simulink model "Li_ion_BatteryPack_Model"  (R2022a)
settings: Solver=VariableStepAuto  StartTime=0.0  StopTime=350  RelTol=1e-3
values from neighbouring files (symbols this model uses):
  A = [0 0 0 ... (first row only)    [Lithium_ion_oneCell_Modeling_continuous_Linear.m]    (also in Lithium_ion_oneCell_Modeling_continuous_new.m)
  A_pack = [A1 zeros(3,9);zeros(3,3) A2 zeros(3,6);zeros(3,6) A3 zeros(3,3);zeros(3,9) A4]    [Lithium_ion_oneCell_Modeling_continuous_new.m]
  A_pack_d = sys_d_pack.A    [Lithium_ion_oneCell_Modeling_continuous_new.m]
  B = [-eta/C_max ... (first row only)    [Lithium_ion_oneCell_Modeling_continuous_Linear.m]    (also in Lithium_ion_oneCell_Modeling_continuous_new.m)
  B_pack = [B1;B2;B3;B4]    [Lithium_ion_oneCell_Modeling_continuous_new.m]
  B_pack_d = sys_d_pack.B    [Lithium_ion_oneCell_Modeling_continuous_new.m]
  R0 = 43e-3    (= 0.043)    [Lithium_ion_oneCell_Modeling_continuous_Linear.m]    (also in Lithium_ion_oneCell_Modeling_continuous_new.m)
  R0_pack = [R0;R0;R0;R0]    [Lithium_ion_oneCell_Modeling_continuous_new.m]
  X10 = [0.6;0;0]    [Lithium_ion_oneCell_Modeling_continuous_new.m]
  Zeta0 = [X10;X20;X30;X40]    [Lithium_ion_oneCell_Modeling_continuous_new.m]
undefined symbols (not defined in the file or in its folder): sigbuilder_block
settings Model: Creator=Asus  LastModifiedBy=Asus

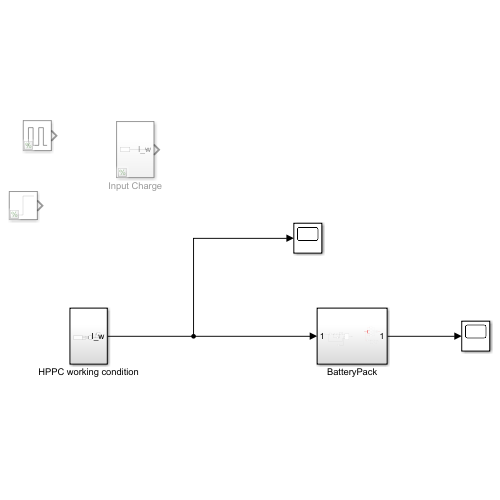
[thumbnail: Simulink's stored preview of the top-level diagram]
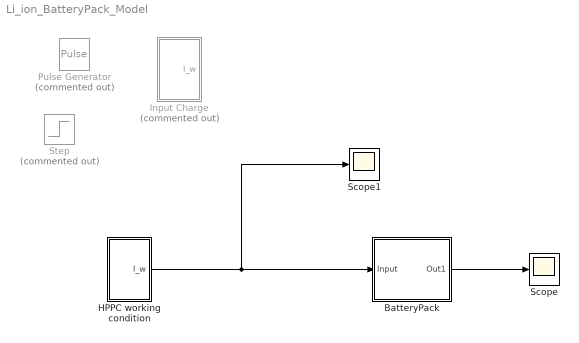
== system Li_ion_BatteryPack_Model ==
  BatteryPack : Subsystem
  HPPC working condition : Subsystem
  Input Charge : Subsystem  Commented=on
  Pulse Generator : DiscretePulseGenerator  Commented=on  PulseType=Time based  Amplitude=-2.4  Period=0.05  PulseWidth=99
  Scope : Scope
  Scope1 : Scope
  Step : Step  Commented=on  Time=10000  Before=-1.2  After=-1.2  SampleTime=0
  wires:
  HPPC working condition/1(I_w) -> Scope1/1, BatteryPack/1(Input)
  BatteryPack/1(Out1) -> Scope/1

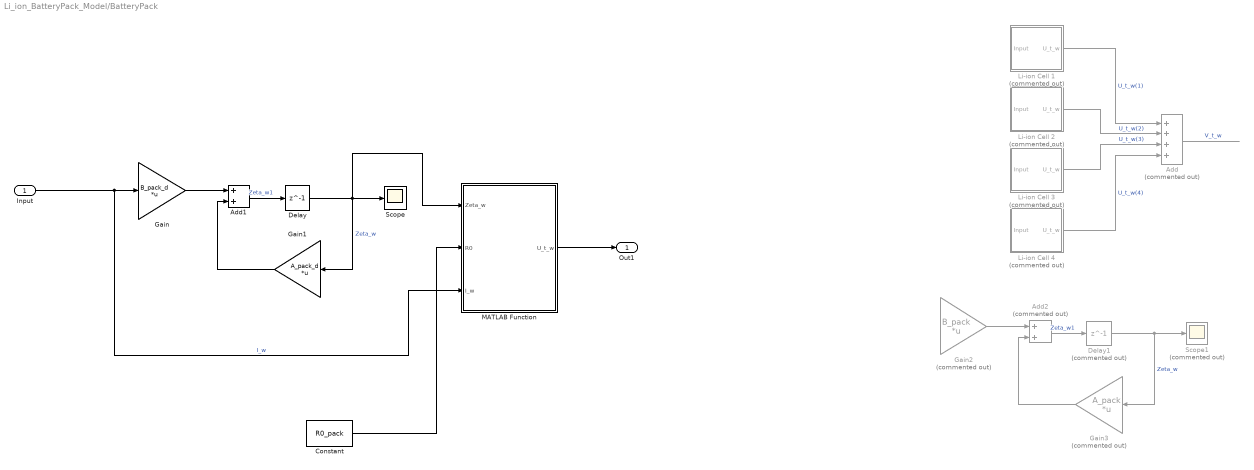
== system Li_ion_BatteryPack_Model/BatteryPack ==
  Input : Inport
  Add : Sum  Commented=on  Inputs=++++
  Add1 : Sum
  Add2 : Sum  Commented=on
  Constant : Constant  Value=R0_pack
  Delay : Delay  DelayLength=1  InitialCondition=Zeta0
  Delay1 : Delay  Commented=on  DelayLength=1  InitialCondition=Zeta0
  Gain : Gain  Gain=B_pack_d  Multiplication=Matrix(K*u)
  Gain1 : Gain  Gain=A_pack_d  Multiplication=Matrix(K*u)
  Gain2 : Gain  Commented=on  Gain=B_pack  Multiplication=Matrix(K*u)
  Gain3 : Gain  Commented=on  Gain=A_pack  Multiplication=Matrix(K*u)
  Li-ion Cell 1 : Subsystem  Commented=on
  Li-ion Cell 2 : Subsystem  Commented=on
  Li-ion Cell 3 : Subsystem  Commented=on
  Li-ion Cell 4 : Subsystem  Commented=on
  MATLAB Function : MATLAB Function  TreatAsAtomicUnit=on
  Scope : Scope
  Scope1 : Scope  Commented=on
  Out1 : Outport
  wires:
  Input/1 -> MATLAB Function/3(I_w), Gain/1  "I_w"
  Gain/1 -> Add1/1
  Add1/1 -> Delay/1  "Zeta_w1"
  Gain1/1 -> Add1/2
  Delay/1 -> Gain1/1, MATLAB Function/1(Zeta_w), Scope/1  "Zeta_w"
  Constant/1 -> MATLAB Function/2(R0)
  MATLAB Function/1(U_t_w) -> Out1/1
  Gain2/1 -> Add2/1
  Delay1/1 -> Scope1/1, Gain3/1  "Zeta_w"
  Li-ion Cell 4/1(U_t_w) -> Add/4  "U_t_w(4)"
  Li-ion Cell 3/1(U_t_w) -> Add/3  "U_t_w(3)"
  Gain3/1 -> Add2/2
  Li-ion Cell 1/1(U_t_w) -> Add/1  "U_t_w(1)"
  ? -> Gain2/1, Li-ion Cell 2/1(Input), Li-ion Cell 1/1(Input), Li-ion Cell 4/1(Input), Li-ion Cell 3/1(Input)  "I_w"
  Li-ion Cell 2/1(U_t_w) -> Add/2  "U_t_w(2)"
  Add/1 -> ?  "V_t_w"
  Add2/1 -> Delay1/1  "Zeta_w1"

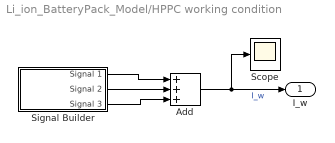
== system Li_ion_BatteryPack_Model/HPPC working condition ==
  Add : Sum  Inputs=+++
  Scope : Scope
  Signal Builder : Subsystem  Tag=STV Subsys  LoadFcn=sigbuilder_block('load');  StartFcn=sigbuilder_block('start');  StopFcn=sigbuilder_block('stop');  ClipboardFcn=sigbuilder_block('clipboard');  mask(Sigbuilder block){tuvar=[0:10]}
      mask help: Simulink:masks:SigbuilderBlock_MD
      mask init:
      | if ~strcmp(get_param(bdroot(gcbh),'SimulationStatus'),'stopped') tuvar = sigbuilder_block('maskInit'); end
      settings: CopyFcn=sigbuilder_block('copy');  DeleteFcn=sigbuilder_block('delete');  ModelCloseFcn=sigbuilder_block('modelClose');  PreSaveFcn=sigbuilder_block('preSave');  PauseFcn=sigbuilder_block('pause');  ContinueFcn=sigbuilder_block('continue');  NameChangeFcn=sigbuilder_block('namechange');  OpenFcn=sigbuilder_block('open',[5.4 36 1141.2 516.6 ]);  CloseFcn=sigbuilder_block('close');
      mask Display: plot(0, 0, 100, 100,[2, 2, 32, 32, 2], [68, 8, 8, 68, 68],[32, 2], [38, 38], [32, 19, 2],[53, 60, 44], [32, 17, 17, 2],[16, 16, 31, 31]);txt = getActiveGroup(gcbh);text(2, 100, txt,'verticalAlignment', 'top');
  I_w : Outport
  wires:
  Add/1 -> Scope/1, I_w/1  "I_w"
  Signal Builder/2(Signal 2) -> Add/2
  Signal Builder/1(Signal 1) -> Add/1
  Signal Builder/3(Signal 3) -> Add/3

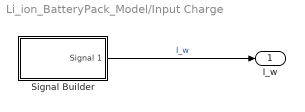
== system Li_ion_BatteryPack_Model/Input Charge ==
  Signal Builder : Subsystem  Tag=STV Subsys  LoadFcn=sigbuilder_block('load');  StartFcn=sigbuilder_block('start');  StopFcn=sigbuilder_block('stop');  ClipboardFcn=sigbuilder_block('clipboard');  mask(Sigbuilder block){tuvar=[0:10]}
      mask help: Simulink:masks:SigbuilderBlock_MD
      mask init:
      | if ~strcmp(get_param(bdroot(gcbh),'SimulationStatus'),'stopped') tuvar = sigbuilder_block('maskInit'); end
      settings: CopyFcn=sigbuilder_block('copy');  DeleteFcn=sigbuilder_block('delete');  ModelCloseFcn=sigbuilder_block('modelClose');  PreSaveFcn=sigbuilder_block('preSave');  PauseFcn=sigbuilder_block('pause');  ContinueFcn=sigbuilder_block('continue');  NameChangeFcn=sigbuilder_block('namechange');  OpenFcn=sigbuilder_block('open',[5.4 36 1141.2 516.6 ]);  CloseFcn=sigbuilder_block('close');
      mask Display: plot(0, 0, 100, 100,[2, 2, 32, 32, 2], [68, 8, 8, 68, 68],[32, 2], [38, 38], [32, 19, 2],[53, 60, 44], [32, 17, 17, 2],[16, 16, 31, 31]);txt = getActiveGroup(gcbh);text(2, 100, txt,'verticalAlignment', 'top');
  I_w : Outport
  wires:
  Signal Builder/1(Signal 1) -> I_w/1  "I_w"

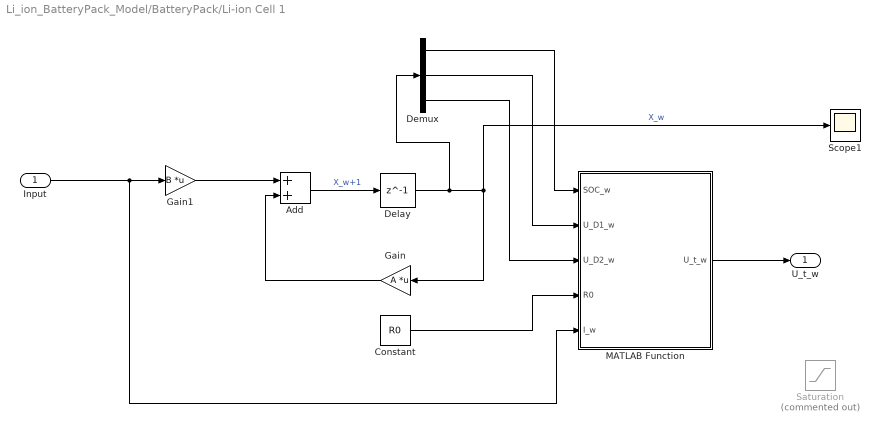
== system Li_ion_BatteryPack_Model/BatteryPack/Li-ion Cell 1 ==
  Input : Inport
  Add : Sum
  Constant : Constant  Value=R0
  Delay : Delay  DelayLength=1  InitialCondition=X10
  Demux : Demux  Outputs=3
  Gain : Gain  Gain=A  Multiplication=Matrix(K*u)
  Gain1 : Gain  Gain=B  Multiplication=Matrix(K*u)
  MATLAB Function : MATLAB Function  TreatAsAtomicUnit=on
  Saturation : Saturate  Commented=on  UpperLimit=4.2  LowerLimit=3
  Scope1 : Scope
  U_t_w : Outport
  wires:
  Input/1 -> MATLAB Function/5(I_w), Gain1/1
  Add/1 -> Delay/1  "X_w+1"
  Demux/1 -> MATLAB Function/1(SOC_w)
  Delay/1 -> Demux/1, Gain/1, Scope1/1  "X_w"
  Gain1/1 -> Add/1
  Demux/3 -> MATLAB Function/3(U_D2_w)
  Gain/1 -> Add/2
  Demux/2 -> MATLAB Function/2(U_D1_w)
  Constant/1 -> MATLAB Function/4(R0)
  MATLAB Function/1(U_t_w) -> U_t_w/1

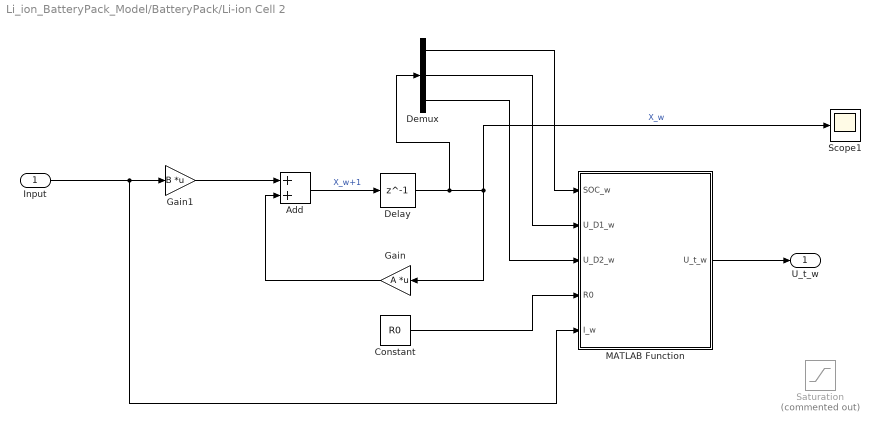
== system Li_ion_BatteryPack_Model/BatteryPack/Li-ion Cell 2 ==
  Input : Inport
  Add : Sum
  Constant : Constant  Value=R0
  Delay : Delay  DelayLength=1  InitialCondition=X10
  Demux : Demux  Outputs=3
  Gain : Gain  Gain=A  Multiplication=Matrix(K*u)
  Gain1 : Gain  Gain=B  Multiplication=Matrix(K*u)
  MATLAB Function : MATLAB Function  TreatAsAtomicUnit=on
  Saturation : Saturate  Commented=on  UpperLimit=4.2  LowerLimit=3
  Scope1 : Scope
  U_t_w : Outport
  wires:
  Input/1 -> MATLAB Function/5(I_w), Gain1/1
  Add/1 -> Delay/1  "X_w+1"
  Demux/1 -> MATLAB Function/1(SOC_w)
  Delay/1 -> Demux/1, Gain/1, Scope1/1  "X_w"
  Gain1/1 -> Add/1
  Demux/3 -> MATLAB Function/3(U_D2_w)
  Gain/1 -> Add/2
  Demux/2 -> MATLAB Function/2(U_D1_w)
  Constant/1 -> MATLAB Function/4(R0)
  MATLAB Function/1(U_t_w) -> U_t_w/1

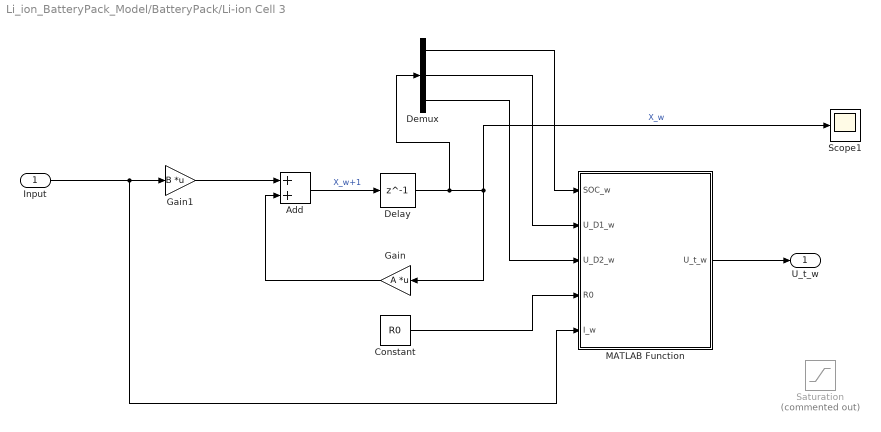
== system Li_ion_BatteryPack_Model/BatteryPack/Li-ion Cell 3 ==
  Input : Inport
  Add : Sum
  Constant : Constant  Value=R0
  Delay : Delay  DelayLength=1  InitialCondition=X10
  Demux : Demux  Outputs=3
  Gain : Gain  Gain=A  Multiplication=Matrix(K*u)
  Gain1 : Gain  Gain=B  Multiplication=Matrix(K*u)
  MATLAB Function : MATLAB Function  TreatAsAtomicUnit=on
  Saturation : Saturate  Commented=on  UpperLimit=4.2  LowerLimit=3
  Scope1 : Scope
  U_t_w : Outport
  wires:
  Input/1 -> MATLAB Function/5(I_w), Gain1/1
  Add/1 -> Delay/1  "X_w+1"
  Demux/1 -> MATLAB Function/1(SOC_w)
  Delay/1 -> Demux/1, Gain/1, Scope1/1  "X_w"
  Gain1/1 -> Add/1
  Demux/3 -> MATLAB Function/3(U_D2_w)
  Gain/1 -> Add/2
  Demux/2 -> MATLAB Function/2(U_D1_w)
  Constant/1 -> MATLAB Function/4(R0)
  MATLAB Function/1(U_t_w) -> U_t_w/1

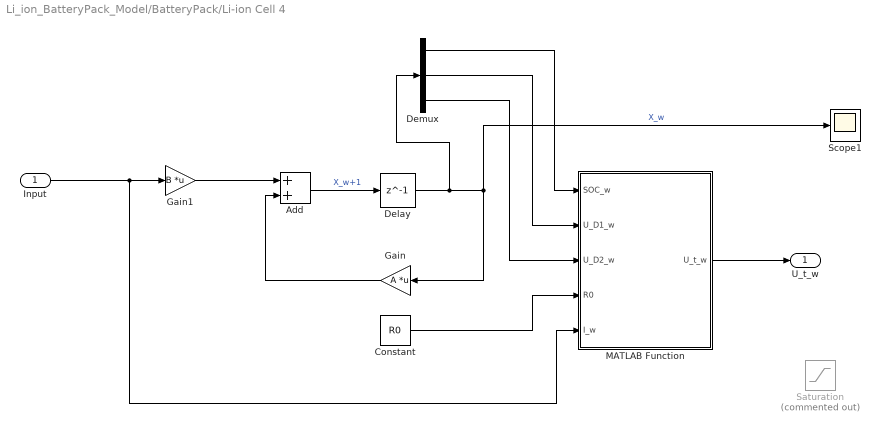
== system Li_ion_BatteryPack_Model/BatteryPack/Li-ion Cell 4 ==
  Input : Inport
  Add : Sum
  Constant : Constant  Value=R0
  Delay : Delay  DelayLength=1  InitialCondition=X10
  Demux : Demux  Outputs=3
  Gain : Gain  Gain=A  Multiplication=Matrix(K*u)
  Gain1 : Gain  Gain=B  Multiplication=Matrix(K*u)
  MATLAB Function : MATLAB Function  TreatAsAtomicUnit=on
  Saturation : Saturate  Commented=on  UpperLimit=4.2  LowerLimit=3
  Scope1 : Scope
  U_t_w : Outport
  wires:
  Input/1 -> MATLAB Function/5(I_w), Gain1/1
  Add/1 -> Delay/1  "X_w+1"
  Demux/1 -> MATLAB Function/1(SOC_w)
  Delay/1 -> Demux/1, Gain/1, Scope1/1  "X_w"
  Gain1/1 -> Add/1
  Demux/3 -> MATLAB Function/3(U_D2_w)
  Gain/1 -> Add/2
  Demux/2 -> MATLAB Function/2(U_D1_w)
  Constant/1 -> MATLAB Function/4(R0)
  MATLAB Function/1(U_t_w) -> U_t_w/1

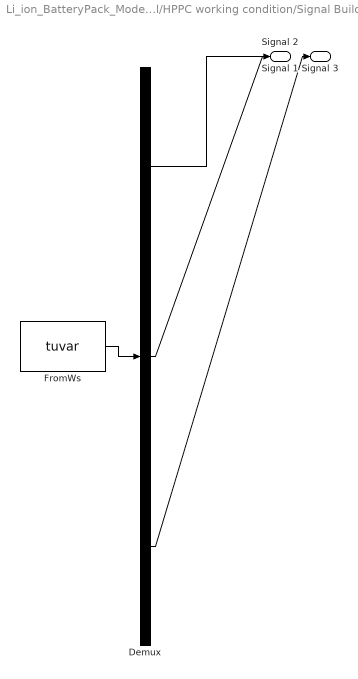
== system Li_ion_BatteryPack_Model/HPPC working condition/Signal Builder ==
  Demux : Demux  Tag=STV Demux  Outputs=3
      settings: DisplayOption=none
  FromWs : FromWorkspace  Tag=STV FromWs  VariableName=tuvar
      SigBuilderData=|
      | common.afterFinalStr = 'Extrapolate'
      | common.sampleTime = 0
      | dataSet.timeRange = [0 350]
      | dataSet.name = 'Group 1'
      | sbobj.Groups.Name = 'Group 1'
      | sbobj.Groups.Signals(1).Name = 'Signal 1'
      | sbobj.Groups.Signals(1).XData = [0 0.1 1 30 30 350]
      | sbobj.Groups.Signals(1).YData = [0 1 4.8 4.8 0 0]
      | sbobj.Groups.Signals(2).Name = 'Signal 2'
      | sbobj.Groups.Signals(2).XData = [0 70 70 80 80 350]
      | sbobj.Groups.Signals(2).YData = [0 0 -2.4 -2.4 1.2 1.2]
      | sbobj.Groups.Signals(3).Name = 'Signal 3'
      | sbobj.Groups.Signals(3).XData = [0 350]
      | sbobj.Groups.Signals(3).YData = [0 0]
      | sbobj.Groups.TimeRange = [0 350]
  Signal 1 : Outport  Tag=STV Outport
  Signal 2 : Outport  Tag=STV Outport  Port=2
  Signal 3 : Outport  Tag=STV Outport  Port=3
  wires:
  FromWs/1 -> Demux/1
  Demux/1 -> Signal 1/1
  Demux/2 -> Signal 2/1
  Demux/3 -> Signal 3/1

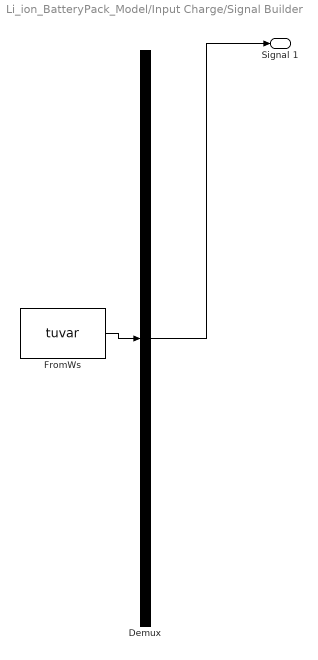
== system Li_ion_BatteryPack_Model/Input Charge/Signal Builder ==
  Demux : Demux  Tag=STV Demux  Outputs=1
      settings: DisplayOption=none
  FromWs : FromWorkspace  Tag=STV FromWs  VariableName=tuvar
      SigBuilderData=|
      | common.afterFinalStr = 'Extrapolate'
      | common.sampleTime = 0
      | dataSet.timeRange = [0 350]
      | dataSet.name = 'Group 1'
      | sbobj.Groups.Name = 'Group 1'
      | sbobj.Groups.Signals.Name = 'Signal 1'
      | sbobj.Groups.Signals.XData = [0 10 10 200 200 350]
      | sbobj.Groups.Signals.YData = [0 0 -2.4 -2.4 0 0]
      | sbobj.Groups.TimeRange = [0 350]
  Signal 1 : Outport  Tag=STV Outport
  wires:
  FromWs/1 -> Demux/1
  Demux/1 -> Signal 1/1

== matlab function Li_ion_BatteryPack_Model/BatteryPack/Li-ion Cell 2/MATLAB Function ==
  data: SOC_w input; U_t_w output; U_D1_w input; U_D2_w input; R0 input; I_w input
function U_t_w = fcn(SOC_w,U_D1_w,U_D2_w,R0,I_w)

p1 = -2744.8612;
p2 = 15237.6802;
p3 = -36711.376;
p4 = 50213.0052;
p5 = -42785.081;
p6 = 23432.4265;
p7 = -8214.5826;
p8 = 1785.199;
p9 = -227.6861;
p10 = 16.3942;
p11 = 3.0665;
f_ocv = p1.*SOC_w.^10 + p2.*SOC_w.^9 + p3.*SOC_w.^8 + p4.*SOC_w.^7 + p5.*SOC_w.^6 + p6.*SOC_w.^5 + p7.*SOC_w.^4 + p8.*SOC_w.^3 + p9.*SOC_w.^2 + p10.*SOC_w + p11;

U_t_w = f_ocv-(U_D1_w+U_D2_w+R0*I_w);

== matlab function Li_ion_BatteryPack_Model/BatteryPack/Li-ion Cell 1/MATLAB Function ==
  data: SOC_w input; U_t_w output; U_D1_w input; U_D2_w input; R0 input; I_w input
function U_t_w = fcn(SOC_w,U_D1_w,U_D2_w,R0,I_w)

p1 = -2744.8612;
p2 = 15237.6802;
p3 = -36711.376;
p4 = 50213.0052;
p5 = -42785.081;
p6 = 23432.4265;
p7 = -8214.5826;
p8 = 1785.199;
p9 = -227.6861;
p10 = 16.3942;
p11 = 3.0665;
f_ocv = p1.*SOC_w.^10 + p2.*SOC_w.^9 + p3.*SOC_w.^8 + p4.*SOC_w.^7 + p5.*SOC_w.^6 + p6.*SOC_w.^5 + p7.*SOC_w.^4 + p8.*SOC_w.^3 + p9.*SOC_w.^2 + p10.*SOC_w + p11;

U_t_w = f_ocv-(U_D1_w+U_D2_w+R0*I_w);

== matlab function Li_ion_BatteryPack_Model/BatteryPack/Li-ion Cell 3/MATLAB Function ==
  data: SOC_w input; U_t_w output; U_D1_w input; U_D2_w input; R0 input; I_w input
function U_t_w = fcn(SOC_w,U_D1_w,U_D2_w,R0,I_w)

p1 = -2744.8612;
p2 = 15237.6802;
p3 = -36711.376;
p4 = 50213.0052;
p5 = -42785.081;
p6 = 23432.4265;
p7 = -8214.5826;
p8 = 1785.199;
p9 = -227.6861;
p10 = 16.3942;
p11 = 3.0665;
f_ocv = p1.*SOC_w.^10 + p2.*SOC_w.^9 + p3.*SOC_w.^8 + p4.*SOC_w.^7 + p5.*SOC_w.^6 + p6.*SOC_w.^5 + p7.*SOC_w.^4 + p8.*SOC_w.^3 + p9.*SOC_w.^2 + p10.*SOC_w + p11;

U_t_w = f_ocv-(U_D1_w+U_D2_w+R0*I_w);

== matlab function Li_ion_BatteryPack_Model/BatteryPack/Li-ion Cell 4/MATLAB Function ==
  data: SOC_w input; U_t_w output; U_D1_w input; U_D2_w input; R0 input; I_w input
function U_t_w = fcn(SOC_w,U_D1_w,U_D2_w,R0,I_w)

p1 = -2744.8612;
p2 = 15237.6802;
p3 = -36711.376;
p4 = 50213.0052;
p5 = -42785.081;
p6 = 23432.4265;
p7 = -8214.5826;
p8 = 1785.199;
p9 = -227.6861;
p10 = 16.3942;
p11 = 3.0665;
f_ocv = p1.*SOC_w.^10 + p2.*SOC_w.^9 + p3.*SOC_w.^8 + p4.*SOC_w.^7 + p5.*SOC_w.^6 + p6.*SOC_w.^5 + p7.*SOC_w.^4 + p8.*SOC_w.^3 + p9.*SOC_w.^2 + p10.*SOC_w + p11;

U_t_w = f_ocv-(U_D1_w+U_D2_w+R0*I_w);

== matlab function Li_ion_BatteryPack_Model/BatteryPack/MATLAB Function ==
  data: Zeta_w input; U_t_w output; R0 input; I_w input
function U_t_w = fcn(Zeta_w,R0,I_w)

% Parameters of SOC function
p1 = -2744.8612;
p2 = 15237.6802;
p3 = -36711.376;
p4 = 50213.0052;
p5 = -42785.081;
p6 = 23432.4265;
p7 = -8214.5826;
p8 = 1785.199;
p9 = -227.6861;
p10 = 16.3942;
p11 = 3.0665;

% Battery Cell 1
R10 = R0(1,1);
SOC1_w = Zeta_w(1,1);
U1_D1_w = Zeta_w(2,1);
U1_D2_w = Zeta_w(3,1);
f1_ocv = p1.*SOC1_w.^10 + p2.*SOC1_w.^9 + p3.*SOC1_w.^8 + p4.*SOC1_w.^7 + p5.*SOC1_w.^6 + p6.*SOC1_w.^5 + p7.*SOC1_w.^4 + p8.*SOC1_w.^3 + p9.*SOC1_w.^2 + p10.*SOC1_w + p11;

% Battery Cell 2
R20 = R0(2,1);
SOC2_w = Zeta_w(4,1);
U2_D1_w = Zeta_w(5,1);
U2_D2_w = Zeta_w(6,1);
f2_ocv = p1.*SOC2_w.^10 + p2.*SOC2_w.^9 + p3.*SOC2_w.^8 + p4.*SOC2_w.^7 + p5.*SOC2_w.^6 + p6.*SOC2_w.^5 + p7.*SOC2_w.^4 + p8.*SOC2_w.^3 + p9.*SOC2_w.^2 + p10.*SOC2_w + p11;

% Battery Cell 3
R30 = R0(3,1);
SOC3_w = Zeta_w(7,1);
U3_D1_w = Zeta_w(8,1);
U3_D2_w = Zeta_w(9,1);
f3_ocv = p1.*SOC3_w.^10 + p2.*SOC3_w.^9 + p3.*SOC3_w.^8 + p4.*SOC3_w.^7 + p5.*SOC3_w.^6 + p6.*SOC3_w.^5 + p7.*SOC3_w.^4 + p8.*SOC3_w.^3 + p9.*SOC3_w.^2 + p10.*SOC3_w + p11;

% Battery Cell 4
R40 = R0(4,1);
SOC4_w = Zeta_w(10,1);
U4_D1_w = Zeta_w(11,1);
U4_D2_w = Zeta_w(12,1);
f4_ocv = p1.*SOC4_w.^10 + p2.*SOC4_w.^9 + p3.*SOC4_w.^8 + p4.*SOC4_w.^7 + p5.*SOC4_w.^6 + p6.*SOC4_w.^5 + p7.*SOC4_w.^4 + p8.*SOC4_w.^3 + p9.*SOC4_w.^2 + p10.*SOC4_w + p11;

U_t_w = ([0 -1 -1]*[SOC1_w;U1_D1_w;U1_D2_w]-R10*I_w+f1_ocv)+([0 -1 -1]*[SOC2_w;U2_D1_w;U2_D2_w]-R20*I_w+f2_ocv)+([0 -1 -1]*[SOC3_w;U3_D1_w;U3_D2_w]-R30*I_w+f3_ocv)+([0 -1 -1]*[SOC4_w;U4_D1_w;U4_D2_w]-R40*I_w+f4_ocv);
